simulink model "vipstaples"  (R2015b)
settings: Solver=FixedStepDiscrete  StartTime=0.0  StopTime=inf  RelTol=1e-3
undefined symbols (not defined in the file or in its folder): gray, strel
libraries: visiontextngfix x4, visionmorphops x2, visionconversions x1, visionstatistics x1, visionsinks x1, vipmisc x1, dspvision x1
settings Model: FPTRunName=Active  ExtModeAutoUpdateStatusClock=off  Creator=The MathWorks, Inc.  LastModifiedBy=The MathWorks, Inc.
settings DataIOCC: SaveFormat=Array  SaveOutput=off  SaveTime=off  SignalLoggingName=logsOut
settings OptimizationCC: ExpressionDepthLimit=2147483647  InitFltsAndDblsToZero=on
settings DebuggingCC: SaveWithParameterizedLinksMsg=none  UnderspecifiedInitializationDetection=Classic  MergeDetectMultiDrivingBlocksExec=none  CheckExecutionContextPreStartOutputMsg=on  CheckExecutionContextRuntimeOutputMsg=on  SignalResolutionControl=TryResolveAllWithWarning  MultiTaskDSMMsg=warning  MultiTaskCondExecSysMsg=none  SigSpecEnsureSampleTimeMsg=none  FcnCallInpInsideContextMsg=UseLocalSettings  StateNameClashWarn=warning  StrictBusMsg=None
settings HardwareCC: ProdBitPerPointer=32  ProdLargestAtomicFloat=None  ProdIntDivRoundTo=Undefined  ProdEndianess=Unspecified  ProdWordSize=32  ProdHWDeviceType=32-bit Generic  TargetBitPerLong=64  TargetBitPerPointer=64  TargetLongLongMode=on  TargetIntDivRoundTo=Zero  TargetEndianess=LittleEndian  TargetWordSize=64  TargetHWDeviceType=Generic->MATLAB Host Computer  ProdEqTarget=off
settings GRTTargetCC: TargetFcnLib=ansi_tfl_tmw.mat  GeneratePreprocessorConditionals=Disable all  CombineOutputUpdateFcns=off  GRTInterface=on
settings ConfigComp: CovModelRefEnable=Off

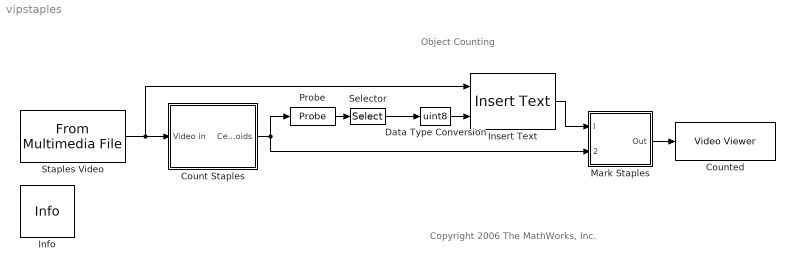
== system vipstaples ==
  note: Object Counting
  note: Copyright 2006 The MathWorks, Inc.
  Count Staples : Subsystem
  Counted : visionsinks/Video Viewer  inputType=Obsolete7b  imagePorts=One multidimensional signal  useColorMap=off  colormapValue=gray(256)  specRange=off  minInputVal=0  maxInputVal=255  FigPos=[372 471 625 348]  AxisZoom=on  trueSizedOnce=on  OpenAtMdlStart=on  DefaultConfigurationName=vipscopes.VideoViewerScopeCfg
  Data Type Conversion : DataTypeConversion  OutDataTypeStr=uint8
  Info : vipmisc/Info  SystemSampleTime=-1
  Insert Text : visiontextngfix/Insert Text  inputType=Obsolete  theText='Staple count: %d'  getTextLocFrom=Specify via dialog  textLoc=[10 280]  getTextColorFrom=Specify via dialog  textColor=255  getTextIntensityFrom=Specify via dialog  textIntensity=255  getTextOpacityFrom=Specify via dialog  textOpacity=1.0  dummyVar2=0  dummyVar3=0  dummyVar4=0  imagePorts=One multidimensional signal  isInputTransposed=off  fontFace=LucidaTypewriterRegular  dummyVar1=0  blockFontSize=30  antiAliased=on
  Mark Staples : Subsystem
  Probe : Probe  ProbeWidth=off  ProbeSampleTime=off  ProbeComplexSignal=off  ProbeSignalDimensions=on  ProbeWidthDataType=uint8
  Selector : Selector  NumberOfDimensions=2  InputPortWidth=3  IndexOptions=Index vector (dialog),Index vector (dialog)  Indices=1,1  OutputSizes=99,1
  Staples Video : dspvision/From Multimedia File  inputFilename=staples.avi  loop=on  numPlays=inf  outputStreams=Video and audio  videoDataType=single  audioDataType=int16  inheritSampleTime=on  userDefinedSampleTime=1/30  noAudioOutput=off  isIntensityVideo=off  fourcc=Intensity  colorVideoFormat=Separate color signals  outputEOF=off  dataOrg=Column-major  audioFrameSize=1024  computeAudioFrameSize=off  outSamplingMode=Frame based
  wires:
  Staples Video/1 -> Insert Text/1, Count Staples/1(Video in)
  Insert Text/1 -> Mark Staples/1(I)
  Count Staples/1(Centroids) -> Probe/1, Mark Staples/2(Centroids)
  Mark Staples/1(Out) -> Counted/1
  Probe/1 -> Selector/1
  Selector/1 -> Data Type Conversion/1
  Data Type Conversion/1 -> Insert Text/2

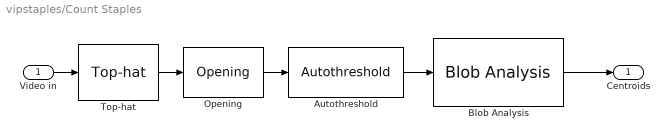
== system vipstaples/Count Staples ==
  Video in : Inport
  Autothreshold : visionconversions/Autothreshold  operator=>  threshOut=off  effMetricOut=off  userDefinedRange=off  umin=0  umax=255  outOfRngOpt=Ignore  scaleThreshold=off  scaleFactor=1  P1Mode=Specify word length  P1WordLength=32  P1FracLength=30  P2Mode=Specify word length  P2WordLength=32  P2FracLength=22  P3Mode=Specify word length  P3WordLength=32  P3FracLength=14  P4Mode=Binary point scaling  P4WordLength=32  P4FracLength=15  Q1Mode=Specify word length  Q1WordLength=32  Q1FracLength=16  EMMode=Specify word length  EMWordLength=16  EMFracLength=14  roundingMode=Floor  overflowMode=off
  Blob Analysis : visionstatistics/Blob Analysis  Tag=vipblks_row_conv  area=off  centroid=on  bBox=off  majorAxis=off  minorAxis=off  angle=off  eccentricity=off  equivDiameterSq=off  extent=off  perimeter=off  maxBlobs=50  warnIfNumBlobsExceeded=on  isCount=off  useMinArea=off  minArea=0  useMaxArea=off  maxArea=inf  excludeBorderBlob=off  outDT=double  isOutVarDim=on  isFill=on  fillValues=-30  conn=8  isLabel=off  outputMode=Binary point scaling  outputWordLength=32  outputFracLength=16  firstCoeffMode=Binary point scaling  firstCoeffWordLength=16  firstCoeffFracLength=14  secondCoeffMode=Binary point scaling  secondCoeffWordLength=32  secondCoeffFracLength=16  accumMode=Binary point scaling  accumWordLength=32  accumFracLength=0  prodOutputMode=Binary point scaling  prodOutputWordLength=32  prodOutputFracLength=16  roundingMode=Floor  overflowMode=off
  Opening : visionmorphops/Opening  nhoodsrc=Specify via dialog  strel=strel('rect',[15 3])
  Top-hat : visionmorphops/Top-hat  imgtype=Intensity  nhoodsrc=Specify via dialog  strel=strel('square',18);
  Centroids : Outport
  wires:
  Blob Analysis/1 -> Centroids/1
  Autothreshold/1 -> Blob Analysis/1
  Opening/1 -> Autothreshold/1
  Top-hat/1 -> Opening/1
  Video in/1 -> Top-hat/1

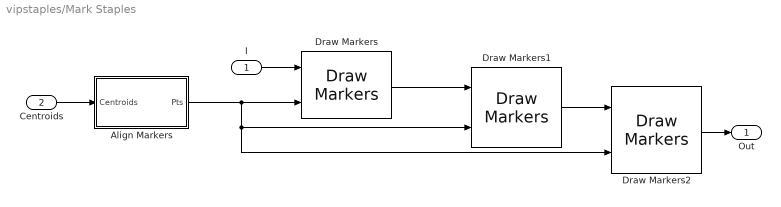
== system vipstaples/Mark Staples ==
  I : Inport
  Centroids : Inport  Port=2
  Align Markers : Subsystem
  Draw Markers : visiontextngfix/Draw Markers  shape=Circle  size=6  fill=off  fillClrSource=Specify via dialog  display=Black  intensity=155  color=[200 120 50]  opacity=1  viewport=Entire image  antialiasing=off  inType=Intensity  imagePorts=One multidimensional signal  prodOutputMode=Binary point scaling  prodOutputWordLength=32  prodOutputFracLength=14  memoryMode=Specify word length  memoryWordLength=16  memoryFracLength=15  roundingMode=Floor  overflowMode=off
  Draw Markers1 : visiontextngfix/Draw Markers  shape=Circle  size=5  fill=off  fillClrSource=Specify via dialog  display=Black  intensity=155  color=[200 120 50]  opacity=1  viewport=Entire image  antialiasing=off  inType=Intensity  imagePorts=One multidimensional signal  prodOutputMode=Binary point scaling  prodOutputWordLength=32  prodOutputFracLength=14  memoryMode=Specify word length  memoryWordLength=16  memoryFracLength=15  roundingMode=Floor  overflowMode=off
  Draw Markers2 : visiontextngfix/Draw Markers  shape=Plus  size=5  fill=off  fillClrSource=Specify via dialog  display=Black  intensity=155  color=[200 120 50]  opacity=1  viewport=Entire image  antialiasing=off  inType=Intensity  imagePorts=One multidimensional signal  prodOutputMode=Binary point scaling  prodOutputWordLength=32  prodOutputFracLength=14  memoryMode=Specify word length  memoryWordLength=16  memoryFracLength=15  roundingMode=Floor  overflowMode=off
  Out : Outport
  wires:
  Centroids/1 -> Align Markers/1(Centroids)
  Align Markers/1(Pts) -> Draw Markers2/2, Draw Markers1/2, Draw Markers/2
  Draw Markers1/1 -> Draw Markers2/1
  Draw Markers/1 -> Draw Markers1/1
  I/1 -> Draw Markers/1
  Draw Markers2/1 -> Out/1

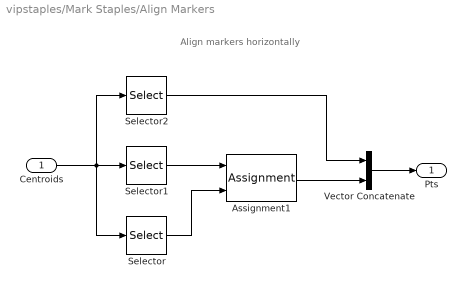
== system vipstaples/Mark Staples/Align Markers ==
  note: Align markers horizontally
  Centroids : Inport
  Assignment1 : Assignment  IndexOptions=Assign all  Indices=1  OutputSizes=1
  Selector : Selector  NumberOfDimensions=2  InputPortWidth=3  IndexOptions=Index vector (dialog),Index vector (dialog)  Indices=1,2  OutputSizes=1,1
  Selector1 : Selector  NumberOfDimensions=2  InputPortWidth=3  IndexOptions=Select all,Index vector (dialog)  Indices=1,2  OutputSizes=1,1
  Selector2 : Selector  NumberOfDimensions=2  InputPortWidth=3  IndexOptions=Select all,Index vector (dialog)  Indices=1,1  OutputSizes=1,1
  Vector Concatenate : Concatenate  Mode=Multidimensional array  ConcatenateDimension=2
  Pts : Outport
  wires:
  Centroids/1 -> Selector/1, Selector1/1, Selector2/1
  Selector/1 -> Assignment1/2
  Selector1/1 -> Assignment1/1
  Selector2/1 -> Vector Concatenate/1
  Assignment1/1 -> Vector Concatenate/2
  Vector Concatenate/1 -> Pts/1
